simulink model "GS"  (R2016a)
settings: Solver=VariableStepAuto  StartTime=0.0  StopTime=10.0  RelTol=1e-3
libraries: simulink x1
settings Model: Creator=Administrator  LastModifiedBy=Administrator

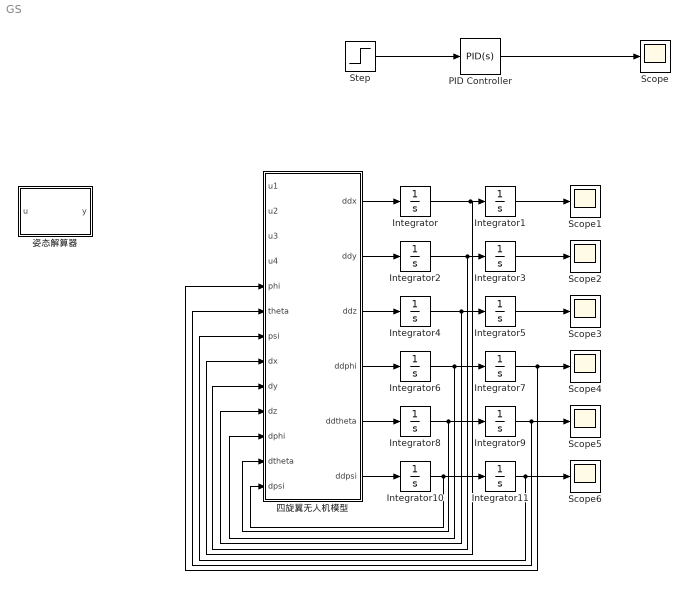
== system GS ==
  Integrator{,1..11} (12 alike) : Integrator
  PID Controller : simulink/Continuous/PID Controller  Controller=PID  TimeDomain=Continuous-time  SampleTime=-1  IntegratorMethod=Forward Euler  FilterMethod=Forward Euler  Form=Parallel  UseFilter=on  ControllerParametersSource=internal  P=1  I=1  D=0  N=100  InitialConditionSource=internal  InitialConditionForIntegrator=0  InitialConditionForFilter=0  ExternalReset=none  LimitOutput=off  UpperSaturationLimit=inf  LowerSaturationLimit=-inf  LinearizeAsGain=on  AntiWindupMode=none  Kb=1  TrackingMode=off  Kt=1  PParamMin=[]  PParamMax=[]  IParamMin=[]  IParamMax=[]  DParamMin=[]  DParamMax=[]  NParamMin=[]  NParamMax=[]  KbParamMin=[]  KbParamMax=[]  KtParamMin=[]  KtParamMax=[]  POutMin=[]  POutMax=[]  IOutMin=[]  IOutMax=[]  DOutMin=[]  DOutMax=[]  NOutMin=[]  NOutMax=[]  KbOutMin=[]  KbOutMax=[]  KtOutMin=[]  KtOutMax=[]  IntegratorOutMin=[]  IntegratorOutMax=[]  FilterOutMin=[]  FilterOutMax=[]  SumOutMin=[]  SumOutMax=[]  SumI1OutMin=[]  SumI1OutMax=[]  SumI2OutMin=[]  SumI2OutMax=[]  SumI3OutMin=[]  SumI3OutMax=[]  SumDOutMin=[]  SumDOutMax=[]  SaturationOutMin=[]  SaturationOutMax=[]  IntegratorContinuousStateAttributes=''  IntegratorStateMustResolveToSignalObject=off  IntegratorRTWStateStorageClass=Auto  FilterContinuousStateAttributes=''  FilterStateMustResolveToSignalObject=off  FilterRTWStateStorageClass=Auto  DifferentiatorICPrevScaledInput=0  DifferentiatorOutMin=[]  DifferentiatorOutMax=[]
  Scope{,1..6} (7 alike) : Scope
  Step : Step  SampleTime=0
  四旋翼无人机模型 : MATLAB Function  TreatAsAtomicUnit=on
  "姿态解算器 " : MATLAB Function  TreatAsAtomicUnit=on
  wires:
  Step/1 -> PID Controller/1
  PID Controller/1 -> Scope/1
  四旋翼无人机模型/1(ddx) -> Integrator/1
  Integrator/1 -> 四旋翼无人机模型/8(dx), Integrator1/1
  Integrator1/1 -> Scope1/1
  四旋翼无人机模型/2(ddy) -> Integrator2/1
  Integrator2/1 -> 四旋翼无人机模型/9(dy), Integrator3/1
  Integrator3/1 -> Scope2/1
  Integrator4/1 -> 四旋翼无人机模型/10(dz), Integrator5/1
  Integrator5/1 -> Scope3/1
  Integrator6/1 -> 四旋翼无人机模型/11(dphi), Integrator7/1
  Integrator7/1 -> 四旋翼无人机模型/5(phi), Scope4/1
  Integrator8/1 -> 四旋翼无人机模型/12(dtheta), Integrator9/1
  Integrator9/1 -> Scope5/1, 四旋翼无人机模型/6(theta)
  Integrator10/1 -> 四旋翼无人机模型/13(dpsi), Integrator11/1
  Integrator11/1 -> Scope6/1, 四旋翼无人机模型/7(psi)
  四旋翼无人机模型/6(ddpsi) -> Integrator10/1
  四旋翼无人机模型/5(ddtheta) -> Integrator8/1
  四旋翼无人机模型/4(ddphi) -> Integrator6/1
  四旋翼无人机模型/3(ddz) -> Integrator4/1

== matlab function GS/姿态解算器  ==
  data: u input; y output
function y = fcn(u)
%#codegen

y = u;

== matlab function GS/四旋翼无人机模型 ==
  data: u1 input; ddx output; u2 input; u3 input; u4 input; phi input; theta input; psi input; dx input; dy input; dz input; dphi input; dtheta input; dpsi input; ddy output; ddz output; ddphi output; ddtheta output; ddpsi output
function [ddx,ddy,ddz,ddphi,ddtheta,ddpsi] = fcn(u1,u2,u3,u4,phi,theta,psi,dx,dy,dz,dphi,dtheta,dpsi)
%%四旋翼无人机参数设置
m = 2; l = 0.2; g = 9.8;
K1 = K2 = K3 = 0.01;
K4 = K5 = K6 = 0.012;
I1 = I2 = I3 = 1.25;
d4 = d5 = d6 = 0.01;

%%动力学方程
ddx = u1(cos(phi)*sin(theta)*cos(psi)+sin(phi)*sin(psi))-K1*dx/m;
ddy = u1(sin(phi)*sin(theta)*cos(psi)-cos(phi)*sin(psi))-K2*dy/m;
ddz = u1*cos(phi)*cos(psi)-g-K3*dz/m;

ddphi = u1-l*K6/I3*dphi;
ddtheta = u2-l*K4/I1*dtheta;
ddpsi = u3 -l*K5/I2*dpsi;


end
